simulink model "Root_Locus_control_model"  (R2019a)
settings: Solver=VariableStepAuto  StartTime=0.0  StopTime=5  MaxStep=0.001  RelTol=1e-3
values from neighbouring files (symbols this model uses):
  TF12 = tfest(data1,2,2)    [TFEXTRACT.m]
libraries: simulink x1
settings Model: Creator=DELL  LastModifiedBy=DELL

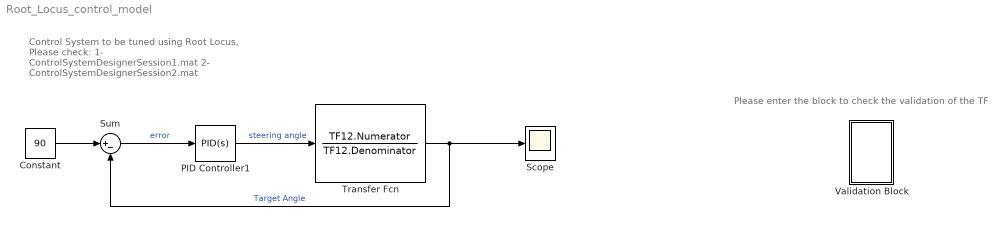
== system Root_Locus_control_model ==
  note: Control System to be tuned using Root Locus,
      | Please check:
      | 1- ControlSystemDesignerSession1.mat
      | 2- ControlSystemDesignerSession2.mat
  note: Please enter the block to check the validation of the TF
  Constant : Constant  Value=90
  PID Controller1 : simulink/Continuous/PID Controller  Controller=PID  Form=Parallel  TimeDomain=Continuous-time  SampleTime=-1  IntegratorMethod=Forward Euler  FilterMethod=Forward Euler  ControllerParametersSource=internal  P=10  I=1000  D=0.001  UseFilter=on  N=100  TunerSelectOption=Transfer Function Based (PID Tuner App)  InitialConditionSource=internal  InitialConditionForIntegrator=0  InitialConditionForFilter=0  DifferentiatorICPrevScaledInput=0  ExternalReset=none  TrackingMode=off  Kt=1  LimitOutput=off  UpperSaturationLimit=inf  LowerSaturationLimit=-inf  LinearizeAsGain=on  AntiWindupMode=none  Kb=1  POutMin=[]  POutMax=[]  IOutMin=[]  IOutMax=[]  DOutMin=[]  DOutMax=[]  NOutMin=[]  NOutMax=[]  SumOutMin=[]  SumOutMax=[]  SaturationOutMin=[]  SaturationOutMax=[]  PParamMin=[]  PParamMax=[]  IParamMin=[]  IParamMax=[]  DParamMin=[]  DParamMax=[]  NParamMin=[]  NParamMax=[]  KbParamMin=[]  KbParamMax=[]  KtParamMin=[]  KtParamMax=[]  KbOutMin=[]  KbOutMax=[]  KtOutMin=[]  KtOutMax=[]  IntegratorOutMin=[]  IntegratorOutMax=[]  FilterOutMin=[]  FilterOutMax=[]  SumI1OutMin=[]  SumI1OutMax=[]  SumI2OutMin=[]  SumI2OutMax=[]  SumI3OutMin=[]  SumI3OutMax=[]  SumI4OutMin=[]  SumI4OutMax=[]  SumDOutMin=[]  SumDOutMax=[]  DifferentiatorOutMin=[]  DifferentiatorOutMax=[]  FilterDiffOutCoefMin=[]  FilterDiffOutCoefMax=[]  ReciprocalOutMin=[]  ReciprocalOutMax=[]  SumDenOutMin=[]  SumDenOutMax=[]  SumNumOutMin=[]  SumNumOutMax=[]  DivideOutMin=[]  DivideOutMax=[]  IntegratorContinuousStateAttributes=''  IntegratorStateMustResolveToSignalObject=off  IntegratorRTWStateStorageClass=Auto  FilterContinuousStateAttributes=''  FilterStateMustResolveToSignalObject=off  FilterRTWStateStorageClass=Auto  ParallelPVariant=InternalParameters  IdealPVariant=Disabled  IVariant=InternalParameters  DVariant=InternalParameters  IntegratorVariant=Continuous  SatVariant=Disabled  AWVariant=Passthrough  PCopyVariant=Disabled  TRVariant=Disabled  FdbkBlocksVariant=Forward  IdealPFdbkVariant=Disabled  SatFdbkVariant=Disabled  DerivativeFilterVariant=ContFilter  NVariant=InternalParameters  NCopyVariant=Disabled  FilterICVariant=InternalICsFilter  IntegratorICVariant=InternalICs  ExternalResetVariant=Disabled  TRSumVariant=Passthrough  SumFdbkVariant=Disabled  SumVariant=Sum_PID
  Scope : Scope
  Sum : Sum  Inputs=|+-
  Transfer Fcn : TransferFcn  Numerator=TF12.Numerator  Denominator=TF12.Denominator
  Validation Block : Subsystem
  wires:
  Sum/1 -> PID Controller1/1  "error"
  Transfer Fcn/1 -> Scope/1, Sum/2  "Target Angle"
  PID Controller1/1 -> Transfer Fcn/1  "steering angle"
  Constant/1 -> Sum/1

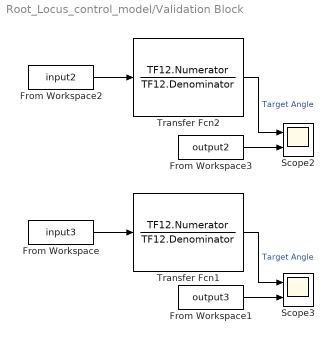
== system Root_Locus_control_model/Validation Block ==
  From Workspace : FromWorkspace  VariableName=input3  SampleTime=0
  From Workspace1 : FromWorkspace  VariableName=output3  SampleTime=0
  From Workspace2 : FromWorkspace  VariableName=input2  SampleTime=0
  From Workspace3 : FromWorkspace  VariableName=output2  SampleTime=0
  "Scope2 " : Scope  NumInputPorts=2
  "Scope3 " : Scope  NumInputPorts=2
  Transfer Fcn1 : TransferFcn  Numerator=TF12.Numerator  Denominator=TF12.Denominator
  Transfer Fcn2 : TransferFcn  Numerator=TF12.Numerator  Denominator=TF12.Denominator
  wires:
  From Workspace/1 -> Transfer Fcn1/1
  Transfer Fcn1/1 -> "Scope3 "/1  "Target Angle"
  Transfer Fcn2/1 -> "Scope2 "/1  "Target Angle"
  From Workspace1/1 -> "Scope3 "/2
  From Workspace2/1 -> Transfer Fcn2/1
  From Workspace3/1 -> "Scope2 "/2
